simulink model "juzhen"  (R2021b)
settings: Solver=VariableStepAuto  StartTime=0.0  StopTime=10.0  RelTol=1e-3
settings Model: Creator=yingguang wang  LastModifiedBy=yingguang wang

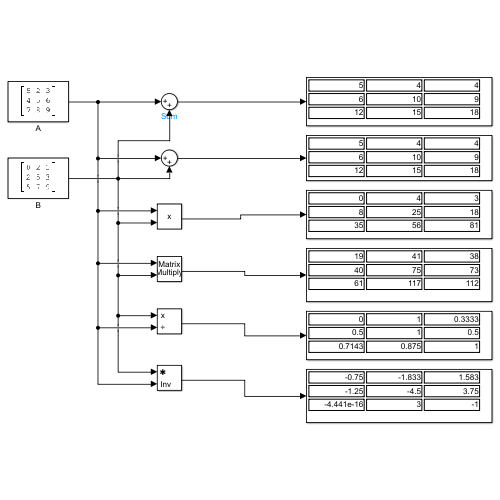
[thumbnail: Simulink's stored preview of the top-level diagram]
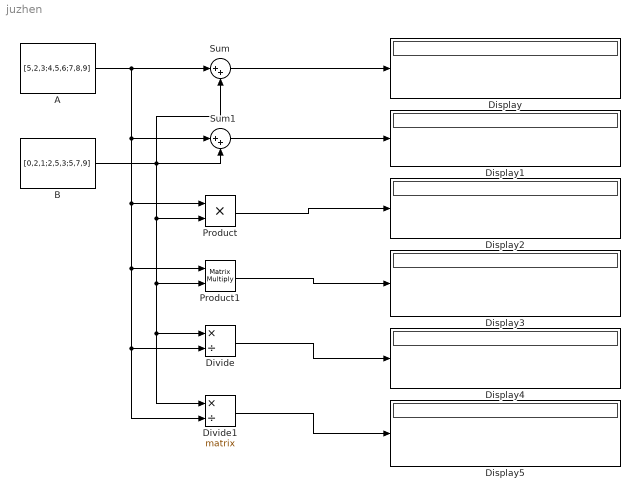
== system juzhen ==
  A : Constant  Value=[5,2,3;4,5,6;7,8,9]
  B : Constant  Value=[0,2,1;2,5,3;5,7,9]
  Display{,1..5} (6 alike) : Display
  Divide : Product  Inputs=*/
  Divide1 : Product  Inputs=*/  Multiplication=Matrix(*)
  Product : Product
  Product1 : Product  Multiplication=Matrix(*)
  Sum : Sum  Inputs=|++
  Sum1 : Sum  Inputs=|++
  wires:
  A/1 -> Divide1/2, Divide/2, Product1/1, Product/1, Sum1/1, Sum/1
  B/1 -> Sum1/2, Product/2, Product1/2, Divide1/1, Divide/1, Sum/2
  Sum/1 -> Display/1
  Sum1/1 -> Display1/1
  Divide/1 -> Display4/1
  Divide1/1 -> Display5/1
  Product1/1 -> Display3/1
  Product/1 -> Display2/1
